simulink model "ME190project1P2"  (R2017a)
settings: Solver=ode5  StartTime=0.0  StopTime=1  FixedStep=0.001  RelTol=1e-3
values from neighbouring files (symbols this model uses):
  A = [zeros(2) eye(2); -inv(M)*K -inv(M)*D]    [project1mat.m]
  B = [0; 0; inv(M)*F]    [project1mat.m]
  C = eye(4)    [project1mat.m]
  DS = [0 0 0 0]'    [project1mat.m]
  IN = [0;(n*3.14/180);0;0]    [project1mat.m]
  K_acker = acker(A,B,P)    [project1mat.m]
settings Model: Creator=kiran  LastModifiedBy=kiran

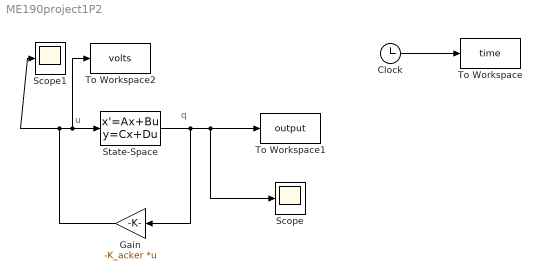
== system ME190project1P2 ==
  note: u
  note: q
  Clock : Clock
  Gain : Gain  Gain=-K_acker  Multiplication=Matrix(K*u)
  Scope : Scope
  Scope1 : Scope
  State-Space : StateSpace  A=A  B=B  C=C  D=DS  X0=IN
  To Workspace : ToWorkspace  VariableName=time  SampleTime=-1
  To Workspace1 : ToWorkspace  VariableName=output  SampleTime=-1
  To Workspace2 : ToWorkspace  VariableName=volts  SampleTime=-1
  wires:
  Clock/1 -> To Workspace/1
  State-Space/1 -> Scope/1, To Workspace1/1, Gain/1
  Gain/1 -> Scope1/1, To Workspace2/1, State-Space/1
